simulink model "profacc_sim"  (R2025b)
settings: Solver=ode45  StartTime=0.0  StopTime=40.0  RelTol=1e-3
settings Model: Creator=sprinkle  LastModifiedBy=sprinkle
settings OptimizationCC: ReuseModelBlockBuffer=off
settings RTWCC: GPUComputeCapability=3.5

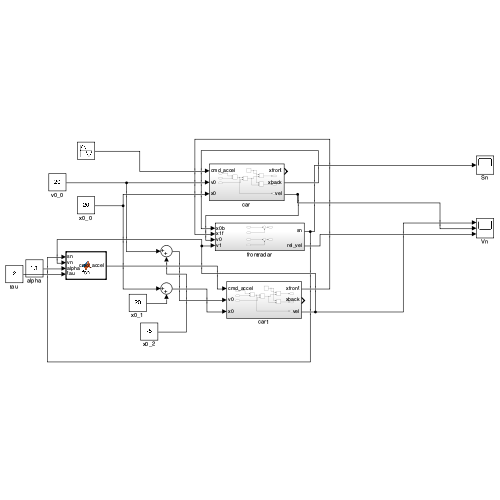
[thumbnail: Simulink's stored preview of the top-level diagram]
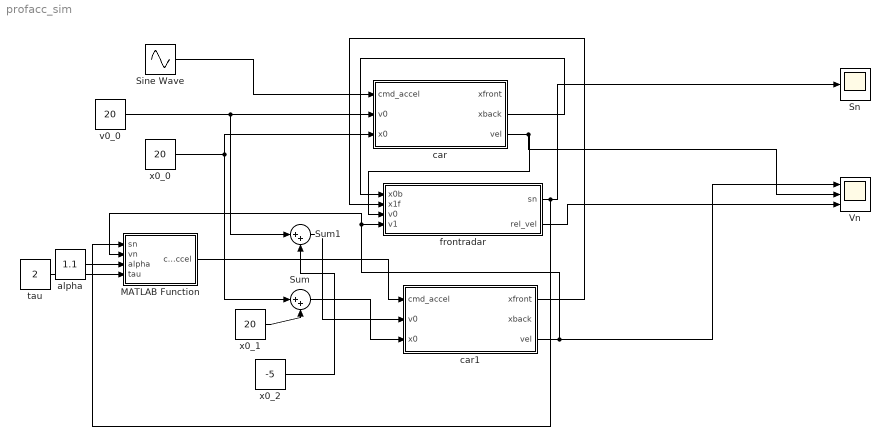
== system profacc_sim ==
  MATLAB Function : MATLAB Function  TreatAsAtomicUnit=on
  Sine Wave : Sin  Amplitude=0.5  SampleTime=0
  Sn : Scope
      settings: ActiveDisplayYMinimum=-1  ActiveDisplayYMaximum=1
  Sum : Sum  Inputs=|++
  Sum1 : Sum  Inputs=|++
  Vn : Scope  NumInputPorts=3
      settings: ActiveDisplayYMinimum=-7.1415088732687861  ActiveDisplayYMaximum=27.260244016990129
  alpha : Constant  Value=1.1
  car : Subsystem
  car1 : Subsystem
  frontradar : Subsystem
  tau : Constant  Value=2
  v0_0 : Constant  Value=20
  x0_0 : Constant  Value=20
  x0_1 : Constant  Value=20
  x0_2 : Constant  Value=-5
  wires:
  Sine Wave/1 -> car/1(cmd_accel)
  tau/1 -> MATLAB Function/4(tau)
  alpha/1 -> MATLAB Function/3(alpha)
  v0_0/1 -> Sum1/1, car/2(v0)
  x0_0/1 -> Sum/1, car/3(x0)
  MATLAB Function/1(cmd_accel) -> car1/1(cmd_accel)
  x0_1/1 -> Sum/2
  Sum/1 -> car1/3(x0)
  x0_2/1 -> Sum1/2
  Sum1/1 -> car1/2(v0)
  car/2(xback) -> frontradar/1(x0b)
  car1/1(xfront) -> frontradar/2(x1f)
  car/3(vel) -> Vn/2, frontradar/3(v0)
  car1/3(vel) -> Vn/1, MATLAB Function/2(vn), frontradar/4(v1)
  frontradar/1(sn) -> Sn/1, MATLAB Function/1(sn)
  frontradar/2(rel_vel) -> Vn/3

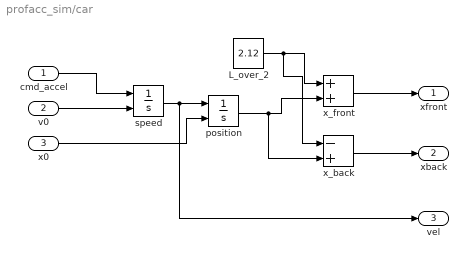
== system profacc_sim/car ==
  cmd_accel : Inport
  v0 : Inport  Port=2
  x0 : Inport  Port=3
  L_over_2 : Constant  Value=2.12
  position : Integrator  InitialConditionSource=external
  speed : Integrator  InitialConditionSource=external
  x_back : Sum  Inputs=-+
  x_front : Sum
  xfront : Outport
  xback : Outport  Port=2
  vel : Outport  Port=3
  wires:
  x_back/1 -> xback/1
  x0/1 -> position/2
  cmd_accel/1 -> speed/1
  speed/1 -> vel/1, position/1
  position/1 -> x_back/2, x_front/2
  x_front/1 -> xfront/1
  v0/1 -> speed/2
  L_over_2/1 -> x_back/1, x_front/1

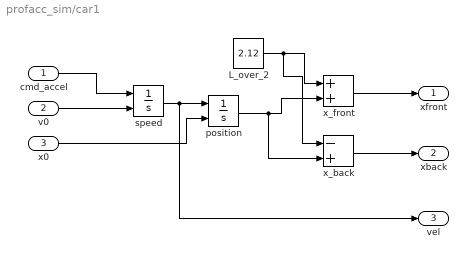
== system profacc_sim/car1 ==
  cmd_accel : Inport
  v0 : Inport  Port=2
  x0 : Inport  Port=3
  L_over_2 : Constant  Value=2.12
  position : Integrator  InitialConditionSource=external
  speed : Integrator  InitialConditionSource=external
  x_back : Sum  Inputs=-+
  x_front : Sum
  xfront : Outport
  xback : Outport  Port=2
  vel : Outport  Port=3
  wires:
  x_back/1 -> xback/1
  x0/1 -> position/2
  cmd_accel/1 -> speed/1
  speed/1 -> vel/1, position/1
  position/1 -> x_back/2, x_front/2
  x_front/1 -> xfront/1
  v0/1 -> speed/2
  L_over_2/1 -> x_back/1, x_front/1

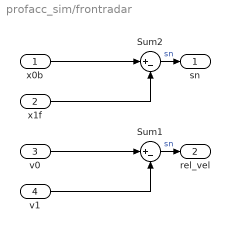
== system profacc_sim/frontradar ==
  x0b : Inport
  x1f : Inport  Port=2
  v0 : Inport  Port=3
  v1 : Inport  Port=4
  Sum1 : Sum  Inputs=|+-
  Sum2 : Sum  Inputs=|+-
  sn : Outport
  rel_vel : Outport  Port=2
  wires:
  x1f/1 -> Sum2/2
  Sum2/1 -> sn/1  "sn"
  x0b/1 -> Sum2/1
  v0/1 -> Sum1/1
  Sum1/1 -> rel_vel/1  "sn"
  v1/1 -> Sum1/2

== matlab function profacc_sim/MATLAB Function ==
  data: sn input; cmd_accel output; vn input; alpha input; tau input
function cmd_accel = fcn(sn,vn,alpha,tau)

cmd_accel = alpha * (sn - tau*vn);
